simulink model "adc_with_impairments_2"  (Simulink 7.4)
settings: Solver=ode45  StartTime=0.0  StopTime=10e-5  RelTol=1e-4
StopFcn:
  | %dt=diff(simout.time);
  | %max_step=max(dt)
  | %min_step = min(dt)
undefined symbols (not defined in the file or in its folder): One, rab_favorites, sided, Subsystem1
libraries: simulink x8, dsparch4 x2, dspsnks4 x2, dspbuff3 x1
settings Model: Creator=dbenson  LastModifiedBy=Dick
settings SolverCC: InitialStep=.1/1e9
settings DataIOCC: Refine=10
settings OptimizationCC: InitFltsAndDblsToZero=on
settings DebuggingCC: SaveWithParameterizedLinksMsg=none  SignalResolutionControl=TryResolveAllWithWarning  MultiTaskDSMMsg=warning  MultiTaskCondExecSysMsg=none  StrictBusMsg=None
settings RTWCC: IncludeERTFirstTime=on
settings GRTTargetCC: TargetFcnLib=ansi_tfl_tmw.mat

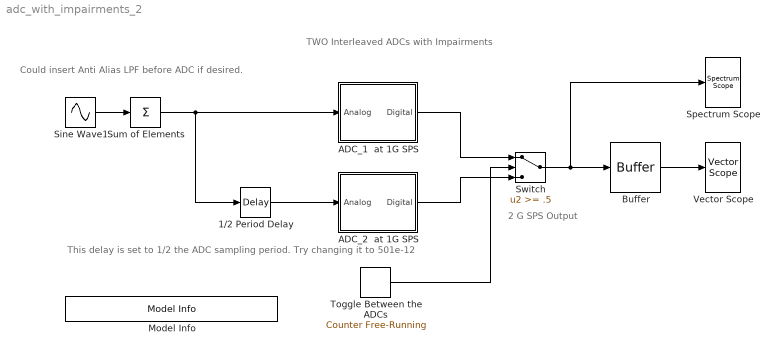
== system adc_with_impairments_2 ==
  note: Could insert Anti Alias LPF
      | before ADC if desired.
  note: TWO Interleaved ADCs with Impairments
  note: This delay is set to 1/2 the ADC sampling period.
      | Try changing it to 501e-12
  note: 2 G SPS Output
  1/2 Period Delay : TransportDelay  DelayTime=500e-12
  ADC_1  at 1G SPS : Subsystem
  ADC_2  at 1G SPS : Subsystem
  Buffer : dspbuff3/Buffer  N=100  V=0  ic=0
  Model Info : simulink/Model-Wide Utilities/Model Info  SystemSampleTime=-1  InitialBlockCM=None  BlockCM=None  Frame=on  DisplayStringWithTags=Copywrite 2005-2010 The MathWorks, Inc.  HorizontalTextAlignment=Center  LeftAlignmentValue=0.5  SourceBlockDiagram=adc_with_impairments_2  TagMaxNumber=20
  Sine Wave1 : Sin  Amplitude=.4  Bias=0  Frequency=2*pi*[20 22]*10e6  Phase=0  Samples=10  SampleTime=0  Offset=0
  Spectrum Scope : dspsnks4/Spectrum Scope  DialogController=dspdialog.SpectrumScope  DialogControllerArgs=DataTag0  SystemSampleTime=-1  ScopeProperties=on  Domain=Frequency  HorizSpan=1  UseBuffer=on  BufferSize=2048  Overlap=0  inpFftLenInherit=off  FFTlength=128  numAvg=2  DisplayProperties=off  AxisGrid=on  Memory=off  FrameNumber=on  AxisLegend=off  AxisZoom=off  OpenScopeAtSimStart=on  OpenScopeImmediately=off  FigPos=[13 485 399 237]  AxisProperties=off  XUnits=Hertz  XRange=One-sided ([0...Fs/2])  XDisplay=0  InheritXIncr=on  XIncr=1.0  XLabel=Samples  XLimit=Auto  YUnits=dBW/Hertz  XMax=1  XMin=0  YLabel=Magnitude-squared, dB  LineProperties=off  wintypeSpecScope=Hann  RsSpecScope=50  betaSpecScope=5  winsampSpecScope=Periodic  XAxisParamsVer=6.8
      settings: YMin=-159.5768  YMax=-66.807
  Sum of Elements : Sum  Inputs=+  OutDataType=sfix(16)  OutScaling=2^-10
  Switch : Switch  Threshold=.5  OutDataType=sfix(16)  OutScaling=2^0
  Toggle Between the ADCs : simulink/Sources/Counter Free-Running  SystemSampleTime=-1  NumBits=1  tsamp=0.5e-9
  Vector Scope : dspsnks4/Vector Scope  DialogController=dspdialog.VectorScope  DialogControllerArgs=DataTag1  ScopeProperties=on  Domain=Time  HorizSpan=1  DisplayProperties=off  AxisGrid=on  Memory=on  FrameNumber=on  AxisLegend=off  AxisZoom=off  OpenScopeAtSimStart=on  OpenScopeImmediately=off  FigPos=[420 485 533 238]  AxisProperties=off  XUnits=Hertz  XRange=[0...Fs/2]  InheritXIncr=on  XIncr=1  XLabel=Time  XLimit=Auto  XMin=0  XMax=1  XStart=0  YUnits=dB  YLabel=Amplitude  LineProperties=off  XAxisParamsVer=6.8
      settings: YMin=-1  YMax=1
  wires:
  Sine Wave1/1 -> Sum of Elements/1
  Sum of Elements/1 -> ADC_1  at 1G SPS/1(Analog), 1/2 Period Delay/1
  1/2 Period Delay/1 -> ADC_2  at 1G SPS/1(Analog)
  Toggle Between the ADCs/1 -> Switch/2
  Switch/1 -> Spectrum Scope/1, Buffer/1
  Buffer/1 -> Vector Scope/1
  ADC_2  at 1G SPS/1(Digital) -> Switch/3
  ADC_1  at 1G SPS/1(Digital) -> Switch/1

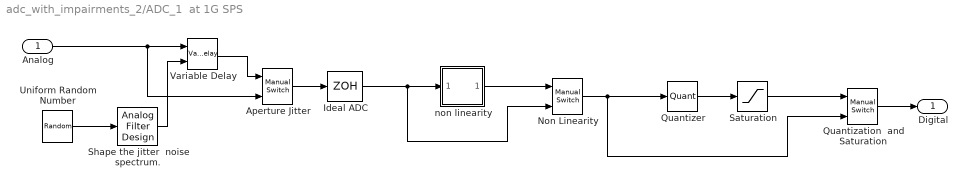
== system adc_with_impairments_2/ADC_1  at 1G SPS ==
  Analog : Inport  OutDataType=sfix(16)  OutScaling=2^0
  Aperture Jitter : simulink/Signal Routing/Manual Switch  SystemSampleTime=-1  sw=0  action=0  varsize=off
  Ideal ADC : ZeroOrderHold  SampleTime=1/1000e6
  Non Linearity : simulink/Signal Routing/Manual Switch  SystemSampleTime=-1  sw=0  action=0  varsize=off
  Quantization  and Saturation : simulink/Signal Routing/Manual Switch  SystemSampleTime=-1  sw=0  action=0  varsize=off
  Quantizer : Quantizer  QuantizationInterval=2^-8
  Saturation : Saturate  UpperLimit=1  LowerLimit=-1
  "Shape the jitter  noise spectrum. " : dsparch4/Analog Filter Design  method=Butterworth  filttype=Lowpass  N=3  Wlo=2*pi*40e6  Whi=80  Rp=2  Rs=40
  Uniform Random Number : UniformRandomNumber  Minimum=0  Maximum=100e-12  Seed=1234  SampleTime=0
  Variable Delay : VariableTransportDelay  MaximumDelay=3e-9  ZeroDelay=on  TransDelayFeedthrough=on
  non linearity : Subsystem  AncestorBlock=rab_favorites/Subsystem1  mask{alpha=.2}
      mask init:
      | x=-3:0.01:3;  y= (1/alpha)*tanh(alpha*x) ;
      mask Display: plot(x,y)
  Digital : Outport  OutDataType=sfix(16)  OutScaling=2^0
  wires:
  Uniform Random Number/1 -> "Shape the jitter  noise spectrum. "/1
  Quantizer/1 -> Saturation/1
  Aperture Jitter/1 -> Ideal ADC/1
  Variable Delay/1 -> Aperture Jitter/1
  Saturation/1 -> Quantization  and Saturation/1
  "Shape the jitter  noise spectrum. "/1 -> Variable Delay/2
  Ideal ADC/1 -> non linearity/1(In1), Non Linearity/2
  non linearity/1(Out1) -> Non Linearity/1
  Non Linearity/1 -> Quantizer/1, Quantization  and Saturation/2
  Analog/1 -> Aperture Jitter/2, Variable Delay/1
  Quantization  and Saturation/1 -> Digital/1

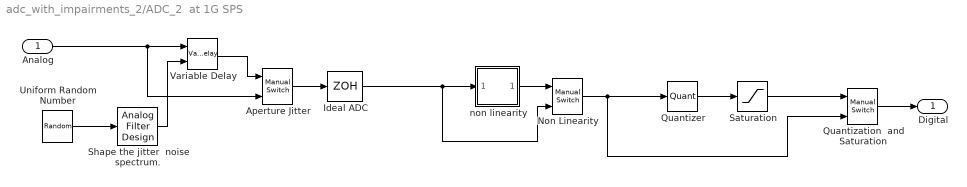
== system adc_with_impairments_2/ADC_2  at 1G SPS ==
  Analog : Inport  OutDataType=sfix(16)  OutScaling=2^0
  Aperture Jitter : simulink/Signal Routing/Manual Switch  SystemSampleTime=-1  sw=0  action=0  varsize=off
  Ideal ADC : ZeroOrderHold  SampleTime=1/1000e6
  Non Linearity : simulink/Signal Routing/Manual Switch  SystemSampleTime=-1  sw=0  action=0  varsize=off
  Quantization  and Saturation : simulink/Signal Routing/Manual Switch  SystemSampleTime=-1  sw=0  action=0  varsize=off
  Quantizer : Quantizer  QuantizationInterval=2^-8
  Saturation : Saturate  UpperLimit=1  LowerLimit=-1
  "Shape the jitter  noise spectrum. " : dsparch4/Analog Filter Design  method=Butterworth  filttype=Lowpass  N=3  Wlo=2*pi*40e6  Whi=80  Rp=2  Rs=40
  Uniform Random Number : UniformRandomNumber  Minimum=0  Maximum=100e-12  Seed=4321  SampleTime=0
  Variable Delay : VariableTransportDelay  MaximumDelay=3e-9  ZeroDelay=on  TransDelayFeedthrough=on
  non linearity : Subsystem  AncestorBlock=rab_favorites/Subsystem1  mask{alpha=.2}
      mask init:
      | x=-3:0.01:3;  y= (1/alpha)*tanh(alpha*x) ;
      mask Display: plot(x,y)
  Digital : Outport  OutDataType=sfix(16)  OutScaling=2^0
  wires:
  Quantization  and Saturation/1 -> Digital/1
  Analog/1 -> Variable Delay/1, Aperture Jitter/2
  Non Linearity/1 -> Quantization  and Saturation/2, Quantizer/1
  non linearity/1(Out1) -> Non Linearity/1
  Ideal ADC/1 -> Non Linearity/2, non linearity/1(In1)
  "Shape the jitter  noise spectrum. "/1 -> Variable Delay/2
  Saturation/1 -> Quantization  and Saturation/1
  Variable Delay/1 -> Aperture Jitter/1
  Aperture Jitter/1 -> Ideal ADC/1
  Quantizer/1 -> Saturation/1
  Uniform Random Number/1 -> "Shape the jitter  noise spectrum. "/1

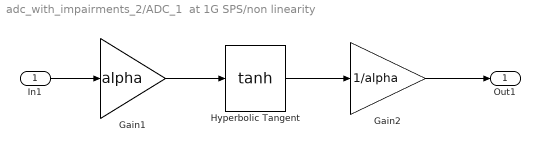
== system adc_with_impairments_2/ADC_1  at 1G SPS/non linearity ==
  In1 : Inport  OutDataType=sfix(16)  OutScaling=2^0
  Gain1 : Gain  Gain=alpha  ParameterDataType=sfix(16)  ParameterScaling=2^0  OutDataType=sfix(16)  OutScaling=2^0  SaturateOnIntegerOverflow=on  OutDataTypeStr=Inherit: Same as input  ParamDataTypeStr=Inherit: Same as input
  Gain2 : Gain  Gain=1/alpha  ParameterDataType=sfix(16)  ParameterScaling=2^0  OutDataType=sfix(16)  OutScaling=2^0  SaturateOnIntegerOverflow=on  OutDataTypeStr=Inherit: Same as input  ParamDataTypeStr=Inherit: Same as input
  Hyperbolic Tangent : Trigonometry  Operator=tanh
  Out1 : Outport  OutDataType=sfix(16)  OutScaling=2^0
  wires:
  Hyperbolic Tangent/1 -> Gain2/1
  In1/1 -> Gain1/1
  Gain2/1 -> Out1/1
  Gain1/1 -> Hyperbolic Tangent/1

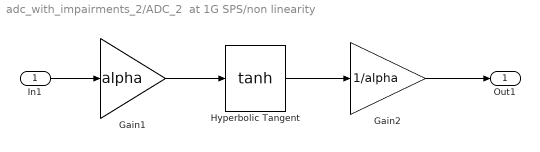
== system adc_with_impairments_2/ADC_2  at 1G SPS/non linearity ==
  In1 : Inport  OutDataType=sfix(16)  OutScaling=2^0
  Gain1 : Gain  Gain=alpha  ParameterDataType=sfix(16)  ParameterScaling=2^0  OutDataType=sfix(16)  OutScaling=2^0  SaturateOnIntegerOverflow=on  OutDataTypeStr=Inherit: Same as input  ParamDataTypeStr=Inherit: Same as input
  Gain2 : Gain  Gain=1/alpha  ParameterDataType=sfix(16)  ParameterScaling=2^0  OutDataType=sfix(16)  OutScaling=2^0  SaturateOnIntegerOverflow=on  OutDataTypeStr=Inherit: Same as input  ParamDataTypeStr=Inherit: Same as input
  Hyperbolic Tangent : Trigonometry  Operator=tanh
  Out1 : Outport  OutDataType=sfix(16)  OutScaling=2^0
  wires:
  Gain1/1 -> Hyperbolic Tangent/1
  Gain2/1 -> Out1/1
  In1/1 -> Gain1/1
  Hyperbolic Tangent/1 -> Gain2/1
